simulink library "csu_tlm_telemetry_lib"  (R2015b)
settings: Solver=ode45  StartTime=0.0  StopTime=10.0  RelTol=1e-3
libraries: util_info_lib x1
settings Model: Creator=mstewart  LastModifiedBy=Mark Agbayani
settings DataIOCC: SaveFormat=Array
settings DebuggingCC: UnderspecifiedInitializationDetection=Classic  MergeDetectMultiDrivingBlocksExec=none  SolverPrmCheckMsg=warning  StateNameClashWarn=warning
settings HardwareCC: ProdBitPerPointer=32  ProdLargestAtomicFloat=None  ProdIntDivRoundTo=Undefined  ProdEndianess=Unspecified  ProdWordSize=32  ProdHWDeviceType=32-bit Generic
settings GRTTargetCC: GeneratePreprocessorConditionals=Disable all
settings ConfigComp: CovModelRefEnable=Off  CovSFcnEnable=off

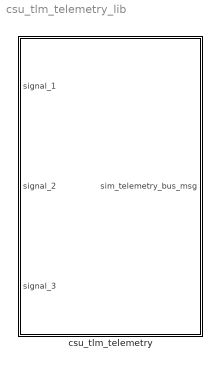
== system csu_tlm_telemetry_lib ==
  csu_tlm_telemetry : Subsystem  mask{num_inputs=3, output_bus_name=sim_telemetry_bus_msg}
      mask prompts: num_inputs "Number of Inputs"; output_bus_name "Bundled Output Bus Name"
      mask init:
      | csu_tlm_telemetry_callback(gcb, num_inputs, output_bus_name);
      mask Display:
      | color('blue');
      | text(0.05, 0.02, 'MoonEx', ...
      |     'HorizontalAlignment', 'Left', ...
      |     'VerticalAlignment', 'Bottom');

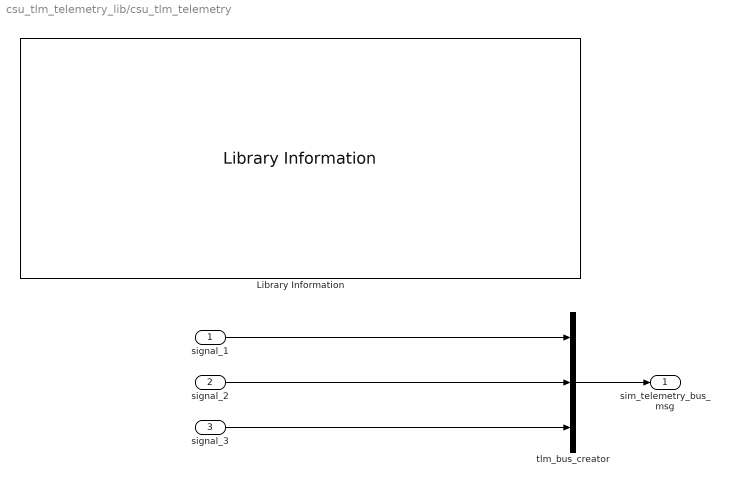
== system csu_tlm_telemetry_lib/csu_tlm_telemetry ==
  signal_1 : Inport
  signal_2 : Inport  Port=2
  signal_3 : Inport  Port=3
  Library Information : util_info_lib/Library Information  owner='NONE'
  tlm_bus_creator : BusCreator  Inputs=3
  sim_telemetry_bus_msg : Outport
  wires:
  signal_3/1 -> tlm_bus_creator/3
  signal_2/1 -> tlm_bus_creator/2
  signal_1/1 -> tlm_bus_creator/1
  tlm_bus_creator/1 -> sim_telemetry_bus_msg/1
